simulink model "SMCobs2int"  (R2015a)
settings: Solver=ode45  StartTime=0.0  StopTime=5  RelTol=1e-3
values from neighbouring files (symbols this model uses):
  A = 1    [setupSMOBS.m]
  alpha1 = 2    [setupSMOBS.m]
  alpha2 = 5    [setupSMOBS.m]
  c = 0.01    [setupSMOBS.m]
  d = 5    [setupSMOBS.m]
  k1 = 70    [setupSMOBS.m]
  k2 = 70    [setupSMOBS.m]
  phi1 = 0.1    [setupSMOBS.m]
  phi2 = 0.005    [setupSMOBS.m]
  x0 = 0    [setupSMOBS.m]
  x1hat0 = 10    [setupSMOBS.m]
  x2hat0 = -10    [setupSMOBS.m]
  xdot0 = 0    [setupSMOBS.m]
settings Model: ExtModeAutoUpdateStatusClock=off  Creator=2414589  LastModifiedBy=rhanz
settings DataIOCC: SignalLoggingSaveFormat=ModelDataLogs
settings OptimizationCC: ExpressionDepthLimit=2147483647  InitFltsAndDblsToZero=on
settings DebuggingCC: SaveWithParameterizedLinksMsg=none  UnderspecifiedInitializationDetection=Classic  MergeDetectMultiDrivingBlocksExec=none  SignalResolutionControl=TryResolveAllWithWarning  SolverPrmCheckMsg=warning  MultiTaskDSMMsg=warning  MultiTaskCondExecSysMsg=none  FcnCallInpInsideContextMsg=UseLocalSettings  StateNameClashWarn=warning
settings GRTTargetCC: TargetFcnLib=ansi_tfl_tmw.mat  CombineOutputUpdateFcns=off  GRTInterface=on

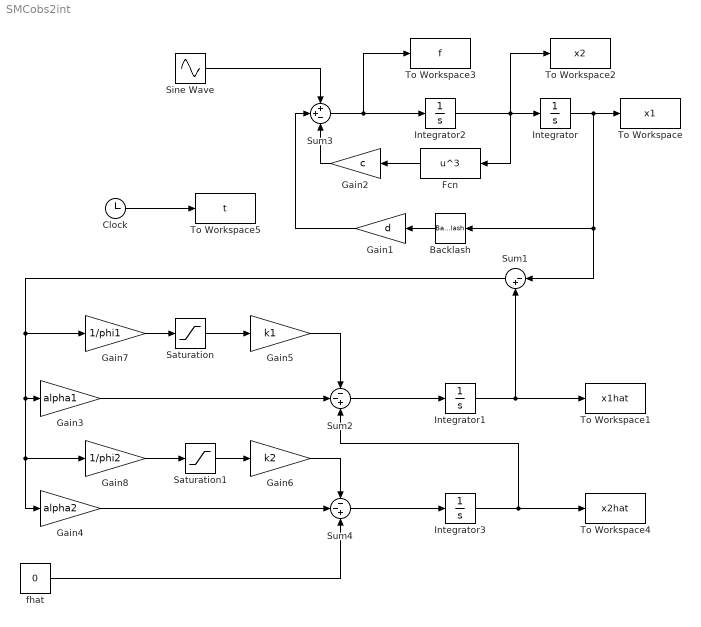
== system SMCobs2int ==
  Backlash : Backlash
  Clock : Clock
  Fcn : Fcn  Expr=u^3
  Gain1 : Gain  Gain=d
  Gain2 : Gain  Gain=c
  Gain3 : Gain  Gain=alpha1
  Gain4 : Gain  Gain=alpha2
  Gain5 : Gain  Gain=k1
  Gain6 : Gain  Gain=k2
  Gain7 : Gain  Gain=1/phi1
  Gain8 : Gain  Gain=1/phi2
  Integrator : Integrator  InitialCondition=x0
  Integrator1 : Integrator  InitialCondition=x1hat0
  Integrator2 : Integrator  InitialCondition=xdot0
  Integrator3 : Integrator  InitialCondition=x2hat0
  Saturation : Saturate  UpperLimit=1  LowerLimit=-1
  Saturation1 : Saturate  UpperLimit=1  LowerLimit=-1
  Sine Wave : Sin  Amplitude=A  SampleTime=0
  Sum1 : Sum  Inputs=|-+
  Sum2 : Sum  Inputs=--+
  Sum3 : Sum  Inputs=++-
  Sum4 : Sum  Inputs=--+
  To Workspace : ToWorkspace  VariableName=x1  SampleTime=-1
  To Workspace1 : ToWorkspace  VariableName=x1hat  SampleTime=-1
  To Workspace2 : ToWorkspace  VariableName=x2  SampleTime=-1
  To Workspace3 : ToWorkspace  VariableName=f  SampleTime=-1
  To Workspace4 : ToWorkspace  VariableName=x2hat  SampleTime=-1
  To Workspace5 : ToWorkspace  VariableName=t  SampleTime=-1
  fhat : Constant  Value=0
  wires:
  Sum2/1 -> Integrator1/1
  Sum3/1 -> To Workspace3/1, Integrator2/1
  Integrator/1 -> Backlash/1, Sum1/1, To Workspace/1
  Backlash/1 -> Gain1/1
  Integrator2/1 -> To Workspace2/1, Fcn/1, Integrator/1
  Fcn/1 -> Gain2/1
  Integrator1/1 -> Sum1/2, To Workspace1/1
  Gain3/1 -> Sum2/2
  Sum1/1 -> Gain7/1, Gain4/1, Gain8/1, Gain3/1
  Gain4/1 -> Sum4/2
  Integrator3/1 -> To Workspace4/1, Sum2/3
  Gain5/1 -> Sum2/1
  Saturation1/1 -> Gain6/1
  Gain6/1 -> Sum4/1
  fhat/1 -> Sum4/3
  Sum4/1 -> Integrator3/1
  Gain1/1 -> Sum3/2
  Gain2/1 -> Sum3/3
  Sine Wave/1 -> Sum3/1
  Gain7/1 -> Saturation/1
  Saturation/1 -> Gain5/1
  Gain8/1 -> Saturation1/1
  Clock/1 -> To Workspace5/1
